simulink model "PIDController"  (R2017b)
settings: Solver=FixedStepDiscrete  StartTime=0.0  StopTime=10  RelTol=1e-3
PreLoadFcn:
  | load('ModelParameters.mat')
StartFcn:
  | Ts=0.03
libraries: simulink x3
settings Model: ExtModeTrigDuration=5  Creator=AlexandrY  LastModifiedBy=Developer
settings SolverCC: AutoInsertRateTranBlk=on
settings DataIOCC: SaveOutput=off  SaveTime=off
settings OptimizationCC: DefaultParameterBehavior=Inlined  UseDivisionForNetSlopeComputation=on  UseFloatMulNetSlope=on  InlineInvariantSignals=on  PassReuseOutputArgsAs=Individual arguments  ZeroExternalMemoryAtStartup=off  ZeroInternalMemoryAtStartup=off  NoFixptDivByZeroProtection=on  EfficientFloat2IntCast=on  LifeSpan=1  MaxStackSize=64
settings DebuggingCC: ParameterTunabilityLossMsg=error  BusObjectLabelMismatch=error
settings HardwareCC: ProdBitPerPointer=32  ProdBitPerSizeT=32  ProdBitPerPtrDiffT=32  ProdLargestAtomicInteger=Long  ProdLargestAtomicFloat=Double  ProdWordSize=32  ProdHWDeviceType=ARM Compatible->ARM Cortex
settings SFSimCC: MATLABDynamicMemAlloc=off
settings RTWCC: SystemTargetFile=ert.tlc  HardwareBoard=NXP FRDM-K64F  PackageGeneratedCodeAndArtifacts=on  PackageName=PIDController  TemplateMakefile=ert_default_tmf  GenerateReport=on  Toolchain=GNU Tools for ARM Embedded Processors  BuildConfiguration=Debug  IncludeHyperlinkInReport=on  LaunchReport=on  GenerateTraceInfo=on  GenerateTraceReport=on  GenerateTraceReportSl=on  GenerateTraceReportSf=on  GenerateTraceReportEml=on  GenerateCodeMetricsReport=on
settings CodeAppCC: ForceParamTrailComments=on  CommentStyle=Single-line  IgnoreCustomStorageClasses=off  OperatorAnnotations=on  SimulinkDataObjDesc=on  SFDataObjDesc=on  MATLABFcnDesc=on  CustomSymbolStrGlobalVar=rt$N$M  CustomSymbolStrType=$N$M  CustomSymbolStrFcn=$N$M$F  CustomSymbolStrMacro=$N$M  InsertBlockDesc=on  StateflowObjectComments=on  MATLABSourceComments=on  EnableCustomComments=on  ReqsInCode=on
settings ERTTargetCC: CodeReplacementLibrary=ARM Cortex-M (Optimized)  MultiwordLength=2048  IncludeMdlTerminateFcn=off  CombineSignalStateStructs=on  SupportAbsoluteTime=off  SupportComplex=off  SupportNonInlinedSFcns=on  ParenthesesLevel=Maximum  InlinedParameterPlacement=NonHierarchical  RootIOFormat=Structure reference  ERTFilePackagingFormat=CompactWithDataFile  ConvertIfToSwitch=off  IndentStyle=Allman

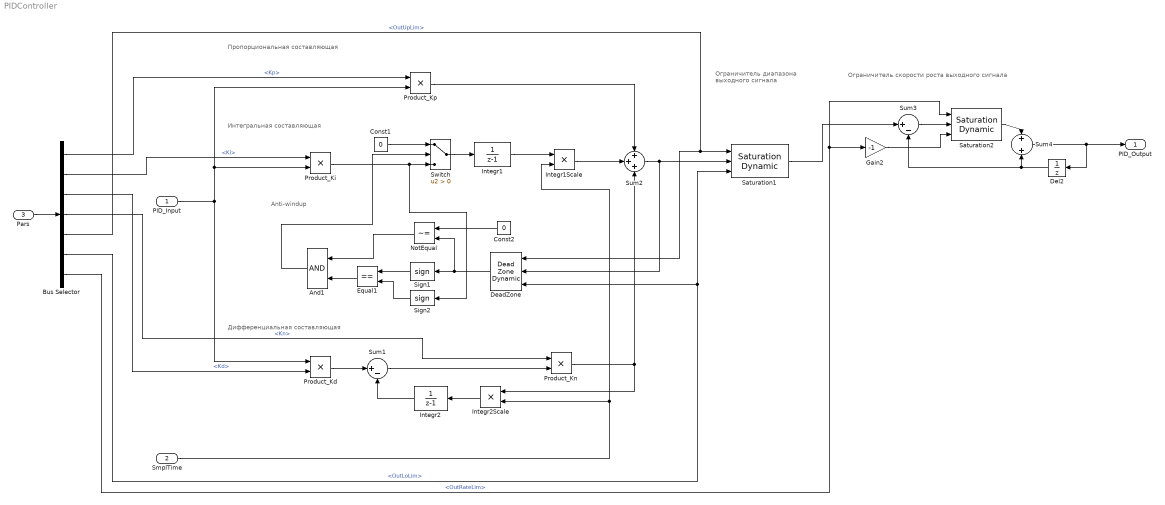
== system PIDController ==
  note: Ограничитель скорости роста выходного сигнала
  note: Пропорциональная составляющая
  note: Интегральная составляющая
  note: Дифференциальная составляющая
  note: Anti-windup
  note: Ограничитель
      | диапазона
      | выходного сигнала
  PID_Input : Inport  OutDataTypeStr=single  PortDimensions=1  SampleTime=[0.029999999999999999,0]
  SmplTime : Inport  Port=2  OutDataTypeStr=single  PortDimensions=1  SampleTime=[0.029999999999999999,0]
  Pars : Inport  Port=3  OutDataTypeStr=Bus: PIDParams  PortDimensions=1  SampleTime=[0.029999999999999999,0]
  And1 : Logic  DisableCoverage=on  OutDataTypeStr=boolean
  Bus Selector : BusSelector  OutputSignals=Kp,Ki,Kd,Kn,OutUpLim,OutLoLim,OutRateLim
  Const1 : Constant  DisableCoverage=on  Value=0  OutDataTypeStr=Inherit: Inherit via back propagation  SampleTime=-1  PreserveConstantTs=on
  Const2 : Constant  Value=0  OutDataTypeStr=Inherit: Inherit via back propagation  SampleTime=-1
  DeadZone : simulink/Discontinuities/Dead Zone Dynamic
      settings: SourceProductName=Simulink  SourceProductBaseCode=SL
  Del2 : UnitDelay  Description=Store in Global RAM  DisableCoverage=on  SampleTime=-1
  Equal1 : RelationalOperator  DisableCoverage=on  Operator===  OutDataTypeStr=boolean  RndMeth=Nearest  InputSameDT=on
  Gain2 : Gain  Gain=-1
  Integr1 : DiscreteTransferFcn  Denominator=[1 -1]
  Integr1Scale : Product
  Integr2 : DiscreteTransferFcn  Denominator=[1 -1]
  Integr2Scale : Product
  NotEqual : RelationalOperator  DisableCoverage=on  Operator=~=  OutDataTypeStr=boolean  RndMeth=Nearest  InputSameDT=on
  Product_Kd : Product
  Product_Ki : Product
  Product_Kn : Product
  Product_Kp : Product
  Saturation1 : simulink/Discontinuities/Saturation Dynamic  OutMin=[]  OutMax=[]  OutDataTypeStr=Inherit: Same as second input  OutDataType=fixdt(1, 16)  OutScaling=2^-10  DoSatur=off
  Saturation2 : simulink/Discontinuities/Saturation Dynamic  OutMin=[]  OutMax=[]  OutDataTypeStr=Inherit: Same as second input  OutDataType=fixdt(1, 16)  OutScaling=2^-10  DoSatur=off
  Sign1 : Signum  DisableCoverage=on
  Sign2 : Signum  DisableCoverage=on
  Sum1 : Sum  Inputs=|+-
  Sum2 : Sum  Inputs=+++
  Sum3 : Sum  Description=Add in CPU  DisableCoverage=on  Inputs=|+-  OutDataTypeStr=Inherit: Inherit via back propagation
  Sum4 : Sum  Description=Add in CPU  OutDataTypeStr=Inherit: Inherit via back propagation
  Switch : Switch  Criteria=u2 > Threshold  InputSameDT=on
  PID_Output : Outport  OutDataTypeStr=single  PortDimensions=1  SampleTime=[0.029999999999999999,0]
  wires:
  Product_Kp/1 -> Sum2/1
  Integr1Scale/1 -> Sum2/2
  Integr2/1 -> Sum1/2
  Sum1/1 -> Product_Kn/2
  Product_Kd/1 -> Sum1/1
  Sum2/1 -> Saturation1/2, DeadZone/2
  Product_Kn/1 -> Integr2Scale/1, Sum2/3
  Const1/1 -> Switch/1
  And1/1 -> Switch/2
  Switch/1 -> Integr1/1
  PID_Input/1 -> Product_Kp/2, Product_Ki/2, Product_Kd/1
  Bus Selector/1 -> Product_Kp/1  "<Kp>"
  Bus Selector/2 -> Product_Ki/1  "<Ki>"
  Bus Selector/3 -> Product_Kd/2  "<Kd>"
  Bus Selector/4 -> Product_Kn/1  "<Kn>"
  Product_Ki/1 -> Switch/3, Sign2/1
  Const2/1 -> NotEqual/1
  DeadZone/1 -> Sign1/1, NotEqual/2
  Sign1/1 -> Equal1/1
  Sign2/1 -> Equal1/2
  NotEqual/1 -> And1/1
  Equal1/1 -> And1/2
  Bus Selector/7 -> Gain2/1, Saturation2/1  "<OutRateLim>"
  SmplTime/1 -> Integr2Scale/2, Integr1Scale/2
  Integr2Scale/1 -> Integr2/1
  Integr1/1 -> Integr1Scale/1
  Pars/1 -> Bus Selector/1
  Bus Selector/5 -> Saturation1/1, DeadZone/1  "<OutUpLim>"
  Bus Selector/6 -> Saturation1/3, DeadZone/3  "<OutLoLim>"
  Sum3/1 -> Saturation2/2
  Saturation1/1 -> Sum3/1
  Gain2/1 -> Saturation2/3
  Saturation2/1 -> Sum4/1
  Del2/1 -> Sum3/2, Sum4/2
  Sum4/1 -> PID_Output/1, Del2/1
